simulink model "example_GroundSourceHX"  (R2018b)
settings: Solver=VariableStepAuto  StartTime=0.0  StopTime=3*24*3600  RelTol=1e-3
libraries: carnot x4
settings Model: Creator=goettsche  LastModifiedBy=drhf

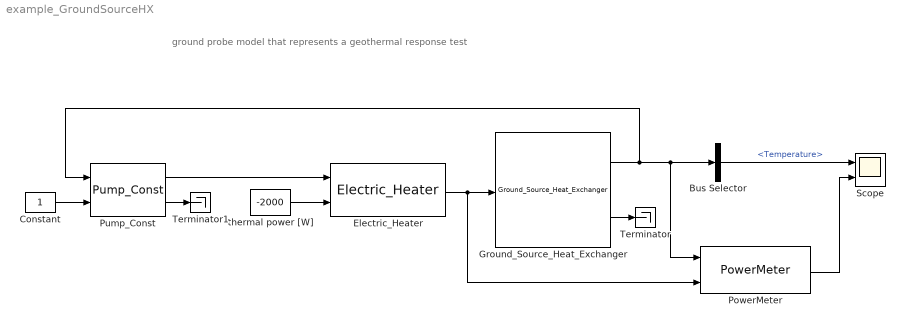
== system example_GroundSourceHX ==
  note: ground probe model that represents a geothermal response test
  Bus Selector : BusSelector  OutputSignals=Temperature
  Constant : Constant
  Electric_Heater : carnot/Source/Boiler/Electric_Heater
      settings: SourceProductName=Carnot
  Ground_Source_Heat_Exchanger : carnot/Source/Heat_Pump/Ground_Source_Heat_Exchanger  Jahresmitteltemp_C=12  TGrad=0.025  lambdaErde=2.0  cpErde=800  rhoErde=2500  lambdaFill=1.0  cpFill=1000  rhoFill=2000  Sondelaenge=100  B=10  Sondendurchmesser=0.032  Bohrdurchmesser=0.18  Bu_param=0.1  sondenfall=1 probe  np=1  DimVert=5  DimRad=10  Gitterfaktor=2.5  LastYear=1
      settings: SourceProductName=Carnot
  PowerMeter : carnot/Control/PowerMeter
      settings: SourceProductName=Carnot
  Pump_Const : carnot/Hydraulics/Pump_Const  mdotmax=1200/3600  dia=0.02  p0=3e5  fluid_id=Water-Glycol Mix  mix=0.25  mix2=0  mix3=0  UA=3  mcp=4182  Tini=20  e0=10  e1=10  e2=-1
      settings: SourceProductName=Carnot
  Scope : Scope  NumInputPorts=2
  Terminator : Terminator
  Terminator1 : Terminator
  thermal power [W] : Constant  Value=-2000
  wires:
  Ground_Source_Heat_Exchanger/1 -> PowerMeter/1, Bus Selector/1, Pump_Const/1
  Bus Selector/1 -> Scope/1  "<Temperature>"
  PowerMeter/1 -> Scope/2
  Ground_Source_Heat_Exchanger/2 -> Terminator/1
  Electric_Heater/1 -> Ground_Source_Heat_Exchanger/1, PowerMeter/2
  thermal power [W]/1 -> Electric_Heater/2
  Pump_Const/1 -> Electric_Heater/1
  Constant/1 -> Pump_Const/2
  Pump_Const/2 -> Terminator1/1
